simulink model "PendoloInverso_LQControl_simulation"  (R2022b)
settings: Solver=VariableStepAuto  StartTime=0.0  StopTime=t_sim  RelTol=1e-3
undefined symbols (not defined in the file): Ac, b1, b2, Bc, deltaT, etag, etam, g, i, K_DLQ, K_LQ, Kgi, km, kt, Lb, Lp, mb, mp, points, Rm, xOrigine
settings Model: Creator=vince  LastModifiedBy=vince

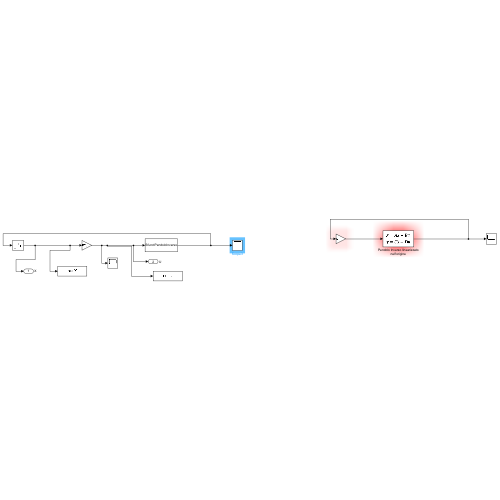
[thumbnail: Simulink's stored preview of the top-level diagram]
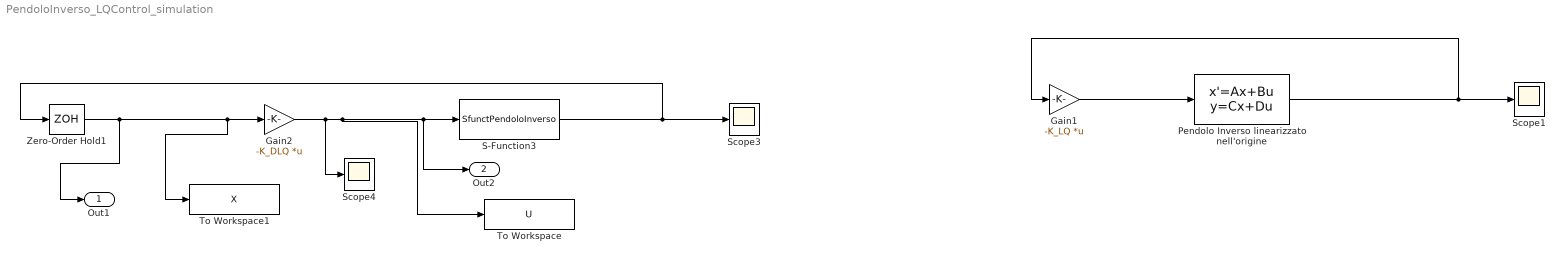
== system PendoloInverso_LQControl_simulation ==
  Gain1 : Gain  Gain=-K_LQ  Multiplication=Matrix(K*u)
  Gain2 : Gain  Gain=-K_DLQ  Multiplication=Matrix(K*u)
  Pendolo Inverso linearizzato nell'origine : StateSpace  A=Ac  B=[Bc]  C=eye(4)  D=[0;0;0;0]  InitialCondition=points{i}-xOrigine  ParameterTunability=Optimized
  S-Function3 : S-Function  FunctionName=SfunctPendoloInverso  Parameters=points{i},mb,mp,Lb,Lp,b1,b2,g,Rm,kt,km,Kgi,etag,etam  SFunctionDeploymentMode=off  EnableBusSupport=off
  Scope1 : Scope
  Scope3 : Scope
  Scope4 : Scope
  To Workspace : ToWorkspace  VariableName=U  SampleTime=-1
  To Workspace1 : ToWorkspace  VariableName=X  SampleTime=-1
  Zero-Order Hold1 : ZeroOrderHold  SampleTime=deltaT
  Out1 : Outport  SignalName=X
  Out2 : Outport  Port=2  SignalName=U
  wires:
  Zero-Order Hold1/1 -> Out1/1, To Workspace1/1, Gain2/1
  Gain2/1 -> To Workspace/1, Out2/1, S-Function3/1, Scope4/1
  S-Function3/1 -> Zero-Order Hold1/1, Scope3/1
  Gain1/1 -> Pendolo Inverso linearizzato nell'origine/1
  Pendolo Inverso linearizzato nell'origine/1 -> Gain1/1, Scope1/1
